simulink model "main_simulation"  (R2025b)
settings: Solver=VariableStepAuto  StartTime=0.0  StopTime=params.sim.duration  MaxStep=params.sim.max_step  MinStep=5  RelTol=0.0001  AbsTol=1e-06
model workspace: external: MAT-File D:\Proiecte Matlab\Cubesat-power-thermal-sim\models\environment\params_simulink.mat (data not in the file)
libraries: fl_lib x5, nesl_utility x4, batteryecm_lib x1
settings Model: Creator=romas  LastModifiedBy=Alex

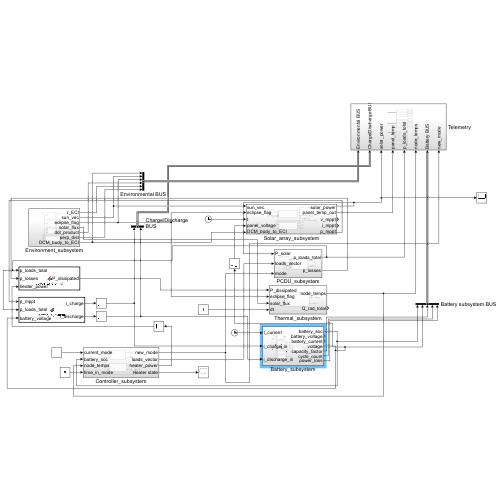
[thumbnail: Simulink's stored preview of the top-level diagram]
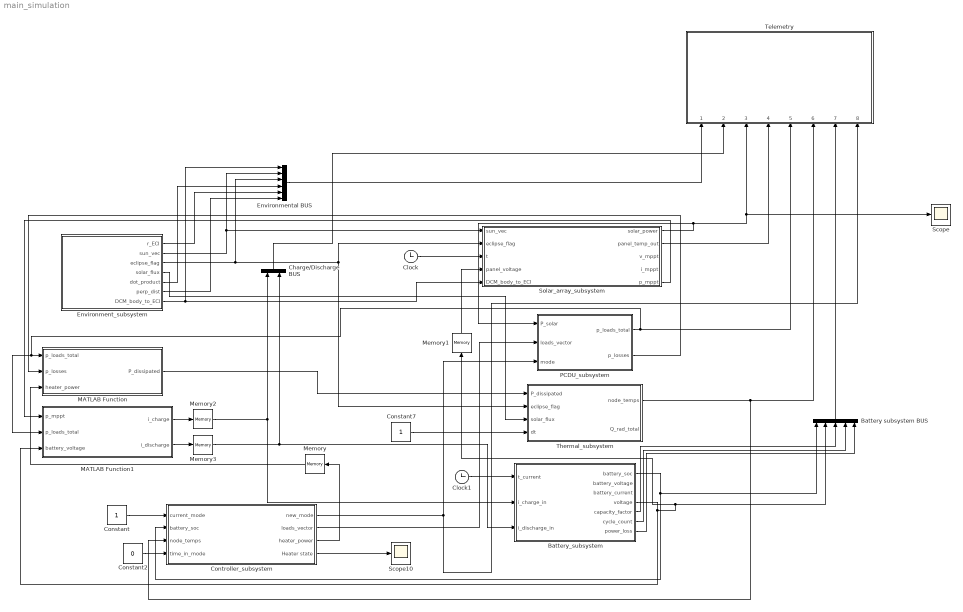
== system main_simulation ==
  Battery subsystem BUS : BusCreator  Inputs=5
  Battery_subsystem : Subsystem
  "Charge/Discharge BUS " : BusCreator  Inputs=2
  Clock : Clock
  Clock1 : Clock
  Constant : Constant
  Constant2 : Constant  Value=0
  Constant7 : Constant
  Controller_subsystem : Subsystem
  Environment_subsystem : Subsystem
  Environmental BUS : BusCreator  Inputs=6
  MATLAB Function : MATLAB Function  TreatAsAtomicUnit=on
  MATLAB Function1 : MATLAB Function  TreatAsAtomicUnit=on
  Memory : Memory
  Memory1 : Memory  InitialCondition=28.8
  Memory2 : Memory
  Memory3 : Memory
  PCDU_subsystem : Subsystem
  Scope : Scope
      settings: ActiveDisplayYMinimum=37.40655674776653  ActiveDisplayYMaximum=42.776597227384748
  Scope10 : Scope
      settings: ActiveDisplayYMinimum=-0.35419792033416531  ActiveDisplayYMaximum=1.2278549732412836  DataLoggingVariableName=ScopeData10
  Solar_array_subsystem : Subsystem
  Telemetry : Subsystem
  Thermal_subsystem : Subsystem
  wires:
  Environment_subsystem/2(sun_vec) -> Solar_array_subsystem/1(sun_vec), Environmental BUS/2
  Environment_subsystem/3(eclipse_flag) -> Environmental BUS/3, Solar_array_subsystem/2(eclipse_flag), Thermal_subsystem/2(eclipse_flag)
  Environment_subsystem/4(solar_flux) -> Thermal_subsystem/3(solar_flux)
  Solar_array_subsystem/1(solar_power) -> PCDU_subsystem/1(P_solar), Scope/1, Telemetry/3(solar_power)
  Constant2/1 -> Controller_subsystem/4(time_in_mode)
  Controller_subsystem/3(heater_power) -> Memory/1
  Controller_subsystem/1(new_mode) -> Telemetry/8(new_mode), PCDU_subsystem/3(mode)
  Controller_subsystem/2(loads_vector) -> PCDU_subsystem/2(loads_vector)
  Battery_subsystem/1(battery_soc) -> Controller_subsystem/2(battery_soc), Battery subsystem BUS/1
  MATLAB Function/1(P_dissipated) -> Thermal_subsystem/1(P_dissipated)
  PCDU_subsystem/1(p_loads_total) -> MATLAB Function1/2(p_loads_total), MATLAB Function/1(p_loads_total), Telemetry/5(p_loads_total)
  PCDU_subsystem/2(p_losses) -> MATLAB Function/2(p_losses)
  Constant7/1 -> Thermal_subsystem/4(dt)
  Memory/1 -> MATLAB Function/3(heater_power)
  Thermal_subsystem/1(node_temps) -> Controller_subsystem/3(node_temps), Telemetry/6(node_temps)
  MATLAB Function1/1(i_charge) -> Memory2/1
  MATLAB Function1/2(i_discharge) -> Memory3/1
  Memory3/1 -> Battery_subsystem/3(i_discharge_in), "Charge/Discharge BUS "/2
  Clock/1 -> Solar_array_subsystem/3(t)
  Clock1/1 -> Battery_subsystem/1(t_current)
  Battery_subsystem/4(voltage) -> Memory1/1, Battery subsystem BUS/2, MATLAB Function1/3(battery_voltage)
  Memory1/1 -> Solar_array_subsystem/4(panel_voltage)
  Memory2/1 -> Battery_subsystem/2(i_charge_in), "Charge/Discharge BUS "/1
  Solar_array_subsystem/2(panel_temp_out) -> Telemetry/4(panel_temp)
  Battery_subsystem/5(capacity_factor) -> Battery subsystem BUS/3
  Battery_subsystem/6(cycle_count) -> Battery subsystem BUS/4
  Battery_subsystem/7(power_loss) -> Battery subsystem BUS/5
  Battery subsystem BUS/1 -> Telemetry/7(Battery BUS)
  Controller_subsystem/4(Heater state) -> Scope10/1
  Environment_subsystem/5(dot_product) -> Environmental BUS/4
  Environment_subsystem/1(r_ECI) -> Environmental BUS/5
  Environment_subsystem/6(perp_dist) -> Environmental BUS/6
  Environmental BUS/1 -> Telemetry/1(Environmental BUS)
  "Charge/Discharge BUS "/1 -> Telemetry/2(Charge/Discharge BUS)
  Environment_subsystem/7(DCM_body_to_ECI) -> Environmental BUS/1, Solar_array_subsystem/5(DCM_body_to_ECI)
  Constant/1 -> Controller_subsystem/1(current_mode)
  Solar_array_subsystem/5(p_mppt) -> MATLAB Function1/1(p_mppt)

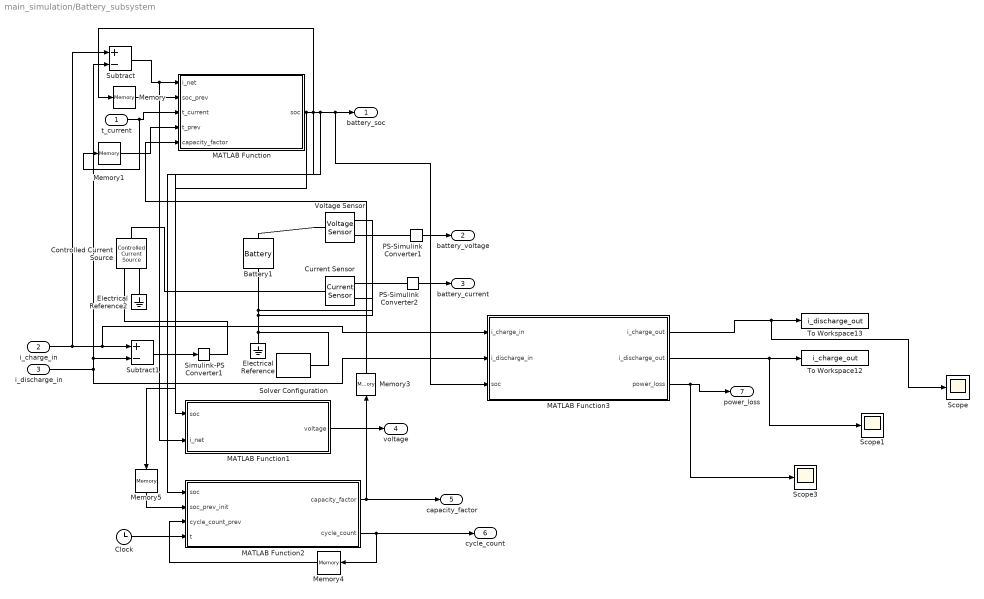
== system main_simulation/Battery_subsystem ==
  t_current : Inport
  i_charge_in : Inport  Port=2
  i_discharge_in : Inport  Port=3
  Battery1 : batteryecm_lib/Battery  Vnom=14.4 V  prm_dir=simscape.enum.battery.prm_dir.disabled  R1_dis=2 Ohm  R1_ch=2 Ohm  R1=0.08 Ohm  prm_AH=simscape.enum.battery.prm_AH.infinite  AH=13.6 A*hr  V1=25.2 V  AH1=2.7 A*hr  prm_R2=simscape.enum.battery.prm_R2.disabled  R2=2000 Ohm  Tmeas=298.15 K  charge_measurement_port=simscape.enum.battery.enable.no  prm_dyn=simscape.enum.battery.prm_dyn.off  Rp1=0.005 Ohm  tau1=30 s  Rp2=0.005 Ohm  tau2=30 s  Rp3=0.005 Ohm  tau3=30 s  Rp4=0.005 Ohm  tau4=30 s  Rp5=0.005 Ohm  tau5=30 s  prm_fade=simscape.enum.battery.prm_fade.disabled  N_fade=100  AH_fade=45 A*hr  R1_fade=2.02 Ohm  R1_ch_fade=2.02 Ohm  V1_fade=10.35 V  prm_age=simscape.enum.battery.prm_age.disabled  prm_age_OCV=simscape.enum.battery.prm_age_OCV.OCV  OCV_age=0.9  SOC_age=60  Tmeas_age=298.15 K  delta_time_age_vec=[0] d  temperature_age_vec=[273] K  OCV_scaling_age=2.2134e6  OCV_offset_age=1.632e6  temp_exp_age=0.515833569 V  t_exp_age=0.75  Vnom_T2=12 V  R1_T2=2.2 Ohm  R1_T2_dis=2.2 Ohm  R1_T2_ch=2.2 Ohm  V1_T2=11.4 V  R2_T2=2200 Ohm  Rp1_T2=0.005 Ohm  tau1_T2=30 s  Rp2_T2=0.005 Ohm  tau2_T2=30 s  Rp3_T2=0.005 Ohm  tau3_T2=30 s  Rp4_T2=0.005 Ohm  tau4_T2=30 s  Rp5_T2=0.005 Ohm  tau5_T2=30 s  Tmeas2=273.15 K  thermal_port=simscape.enum.thermaleffects.omit  thermal_mass=30000 J/K  i_specify=off  i_priority=None  i=0 A  i_nominal_specify=off  i_nominal_value=1  i_nominal_unit=A  v_specify=off  v_priority=None  v=0 V  v_nominal_specify=off  v_nominal_value=1  v_nominal_unit=V  charge_specify=off  charge_priority=High  charge=50 A*hr  charge_nominal_specify=off  charge_nominal_value=1  charge_nominal_unit=A*hr  num_cycles_specify=off  num_cycles_priority=High  num_cycles=0  num_cycles_nominal_specify=off  num_cycles_nominal_value=1  num_cycles_nominal_unit=1  temperature_specify=off  temperature_priority=High  temperature=298.15 K  temperature_nominal_specify=off  temperature_nominal_value=1  temperature_nominal_unit=K
  Clock : Clock
  Controlled Current Source : fl_lib/Electrical/Electrical Sources/Controlled Current Source
      settings: LogSimulationData=on
  Current Sensor : fl_lib/Electrical/Electrical Sensors/Current Sensor
  Electrical Reference : fl_lib/Electrical/Electrical Elements/Electrical Reference
  Electrical Reference2 : fl_lib/Electrical/Electrical Elements/Electrical Reference
  MATLAB Function : MATLAB Function  TreatAsAtomicUnit=on
  MATLAB Function1 : MATLAB Function  TreatAsAtomicUnit=on
  MATLAB Function2 : MATLAB Function  TreatAsAtomicUnit=on
  MATLAB Function3 : MATLAB Function  TreatAsAtomicUnit=on
  Memory : Memory  InitialCondition=0.5
  Memory1 : Memory
  Memory3 : Memory  InitialCondition=1
  Memory4 : Memory
  Memory5 : Memory  InitialCondition=0.5
  PS-Simulink Converter1 : nesl_utility/PS-Simulink Converter  PhysicalDomain=network_engine_domain  SubClassName=ps_output  LeftPortType=input  RightPortType=output  PseudoPeriodic=off  Frequencies=[]  VectorFormat=inherit  Unit=inherit  AffineConversion=off
  PS-Simulink Converter2 : nesl_utility/PS-Simulink Converter  PhysicalDomain=network_engine_domain  SubClassName=ps_output  LeftPortType=input  RightPortType=output  PseudoPeriodic=off  Frequencies=[]  VectorFormat=inherit  Unit=inherit  AffineConversion=off
  Scope : Scope
      settings: ActiveDisplayYMinimum=1.0175731701322981  ActiveDisplayYMaximum=4.0182844452187787  DataLoggingVariableName=ScopeData6
  Scope1 : Scope
      settings: ActiveDisplayYMinimum=-0.49399999999999988  ActiveDisplayYMaximum=4.446  DataLoggingVariableName=ScopeData8
  Scope3 : Scope
      settings: ActiveDisplayYMinimum=-7.2208170321005092  ActiveDisplayYMaximum=9.8697764484998771  DataLoggingVariableName=ScopeData11
  Simulink-PS Converter1 : nesl_utility/Simulink-PS Converter  PhysicalDomain=network_engine_domain  SubClassName=ps_input  LeftPortType=input  RightPortType=output  PseudoPeriodic=off  Frequencies=[]  NoiseDistribution=none  NoiseParameters=[]  Unit=1  AffineConversion=off  FilteringAndDerivatives=provide  SimscapeFilterOrder=1  InputFilterTimeConstant=0.001  UdotUserProvided=0
  Solver Configuration : nesl_utility/Solver Configuration  PhysicalDomain=network_engine_domain  SubClassName=solver  LeftPortType=input  RightPortType=generic  Tones=[]  Harmonics=[]  SimulateNoise=off  Profile=off  UseLocalSampling=off  EnableSwitchedLinearOptims=on  FrequencyDomain=off  UseCCode=off  RelTol=0.001  AbsTol=0.001  MinStep=1e-09  ToWorkspace=off  RevertToSquareIcSolve=off  NumHomotopyIterations=100  PhasorMode=off  PhasorModeNumHarmonics=1  ConsistencySolver=NEWTON_XTOL_AFTER_FTOL  IndexReductionMethod=DerivativeReplacement  DoDC=off  ResidualTolerance=1e-09  ConsistencyTolSource=GLOBAL  ConsistencyAbsTol=0.001  ConsistencyRelTol=0.001  ConsistencyTolFactor=0.001  UseLocalSolver=off  LocalSolverChoice=NE_BACKWARD_EULER_ADVANCER  ResolveIndetEquations=on  FunctionEvalNumThread=1  LocalSolverSampleTime=0.001  DoFixedCost=off  MaxNonlinIter=3  MaxModeIter=2  ComputeImpulses=off  ImpulseIterations=2  LinearAlgebra=auto  LinearAlgebraNumThread=0  EquationFormulation=NE_TIME_EF  DelaysMemoryBudget=1024  AutomaticFiltering=on  FilteringTimeConstant=0.001  PartitionStorageMethod=AS_NEEDED  PartitionMemoryBudget=1024  PartitionMethod=ROBUST  MultibodyUseLocalSolver=off  MultibodyLocalSolverChoice=ODE1  MultibodyLocalSolverSampleTime=0.001
  Subtract : Sum  Inputs=+-
  Subtract1 : Sum  Inputs=+-
  To Workspace12 : ToWorkspace  VariableName=i_charge_out  SaveFormat=Timeseries  SampleTime=-1
  To Workspace13 : ToWorkspace  VariableName=i_discharge_out  SaveFormat=Timeseries  SampleTime=-1
  Voltage Sensor : fl_lib/Electrical/Electrical Sensors/Voltage Sensor
  battery_soc : Outport
  battery_voltage : Outport  Port=2
  battery_current : Outport  Port=3
  voltage : Outport  Port=4
  capacity_factor : Outport  Port=5
  cycle_count : Outport  Port=6
  power_loss : Outport  Port=7
  wires:
  MATLAB Function/1(soc) -> MATLAB Function1/1(soc), Memory5/1, Memory/1, MATLAB Function3/3(soc), battery_soc/1, MATLAB Function2/1(soc)
  Subtract1/1 -> Simulink-PS Converter1/1
  PS-Simulink Converter2/1 -> battery_current/1
  PS-Simulink Converter1/1 -> battery_voltage/1
  t_current/1 -> MATLAB Function/3(t_current), Memory1/1
  Memory1/1 -> MATLAB Function/4(t_prev)
  MATLAB Function1/1(voltage) -> voltage/1
  MATLAB Function2/1(capacity_factor) -> Memory3/1, capacity_factor/1
  Clock/1 -> MATLAB Function2/4(t)
  Memory3/1 -> MATLAB Function/5(capacity_factor)
  MATLAB Function2/2(cycle_count) -> Memory4/1, cycle_count/1
  Memory4/1 -> MATLAB Function2/3(cycle_count_prev)
  Memory/1 -> MATLAB Function/2(soc_prev)
  Memory5/1 -> MATLAB Function2/2(soc_prev_init)
  Subtract/1 -> MATLAB Function1/2(i_net), MATLAB Function/1(i_net)
  i_charge_in/1 -> Subtract/1, MATLAB Function3/1(i_charge_in), Subtract1/1
  i_discharge_in/1 -> MATLAB Function3/2(i_discharge_in), Subtract/2, Subtract1/2
  MATLAB Function3/1(i_charge_out) -> Scope/1, To Workspace13/1
  MATLAB Function3/2(i_discharge_out) -> Scope1/1, To Workspace12/1
  MATLAB Function3/3(power_loss) -> Scope3/1, power_loss/1
  connections:
  Battery1/RConn1 -- Voltage Sensor/RConn2 -- Current Sensor/RConn2 -- Solver Configuration/RConn1 -- Electrical Reference/LConn1
  PS-Simulink Converter1/LConn1 -- Voltage Sensor/RConn1
  PS-Simulink Converter2/LConn1 -- Current Sensor/RConn1
  Simulink-PS Converter1/RConn1 -- Controlled Current Source/RConn1
  Electrical Reference2/LConn1 -- Controlled Current Source/RConn2
  Controlled Current Source/LConn1 -- Current Sensor/LConn1
  Voltage Sensor/LConn1 -- Battery1/LConn1

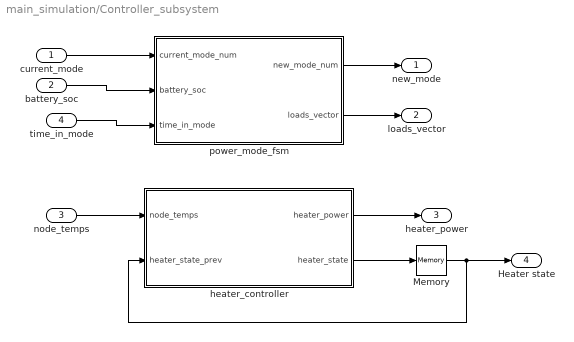
== system main_simulation/Controller_subsystem ==
  current_mode : Inport
  battery_soc : Inport  Port=2
  node_temps : Inport  Port=3
  time_in_mode : Inport  Port=4
  Memory : Memory  InitialCondition=[0;0;0]
  heater_controller : MATLAB Function  TreatAsAtomicUnit=on
  power_mode_fsm : MATLAB Function  TreatAsAtomicUnit=on
  new_mode : Outport
  loads_vector : Outport  Port=2
  heater_power : Outport  Port=3
  Heater state : Outport  Port=4
  wires:
  battery_soc/1 -> power_mode_fsm/2(battery_soc)
  node_temps/1 -> heater_controller/1(node_temps)
  time_in_mode/1 -> power_mode_fsm/3(time_in_mode)
  heater_controller/2(heater_state) -> Memory/1
  power_mode_fsm/2(loads_vector) -> loads_vector/1
  heater_controller/1(heater_power) -> heater_power/1
  Memory/1 -> Heater state/1, heater_controller/2(heater_state_prev)
  power_mode_fsm/1(new_mode_num) -> new_mode/1
  current_mode/1 -> power_mode_fsm/1(current_mode_num)

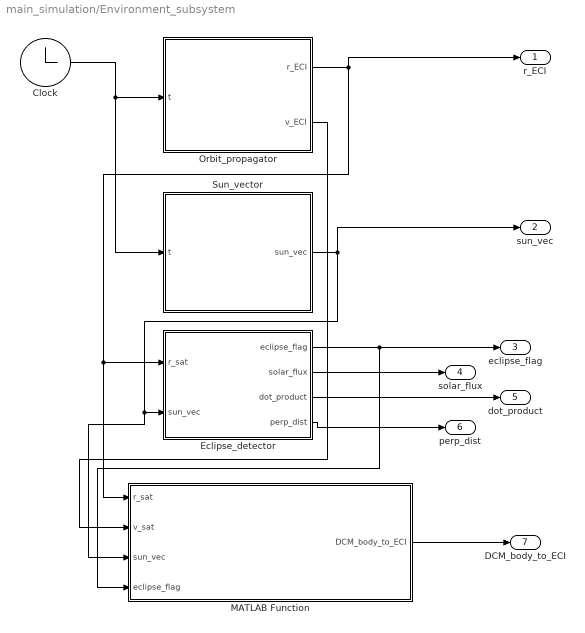
== system main_simulation/Environment_subsystem ==
  Clock : Clock
  Eclipse_detector : MATLAB Function  TreatAsAtomicUnit=on
  MATLAB Function : MATLAB Function  TreatAsAtomicUnit=on
  Orbit_propagator : MATLAB Function  TreatAsAtomicUnit=on
  Sun_vector : MATLAB Function  TreatAsAtomicUnit=on
  r_ECI : Outport
  sun_vec : Outport  Port=2
  eclipse_flag : Outport  Port=3
  solar_flux : Outport  Port=4
  dot_product : Outport  Port=5
  perp_dist : Outport  Port=6
  DCM_body_to_ECI : Outport  Port=7
  wires:
  Clock/1 -> Sun_vector/1(t), Orbit_propagator/1(t)
  Orbit_propagator/1(r_ECI) -> r_ECI/1, MATLAB Function/1(r_sat), Eclipse_detector/1(r_sat)
  Sun_vector/1(sun_vec) -> sun_vec/1, MATLAB Function/3(sun_vec), Eclipse_detector/2(sun_vec)
  Eclipse_detector/1(eclipse_flag) -> MATLAB Function/4(eclipse_flag), eclipse_flag/1
  Eclipse_detector/2(solar_flux) -> solar_flux/1
  Eclipse_detector/3(dot_product) -> dot_product/1
  Eclipse_detector/4(perp_dist) -> perp_dist/1
  Orbit_propagator/2(v_ECI) -> MATLAB Function/2(v_sat)
  MATLAB Function/1(DCM_body_to_ECI) -> DCM_body_to_ECI/1

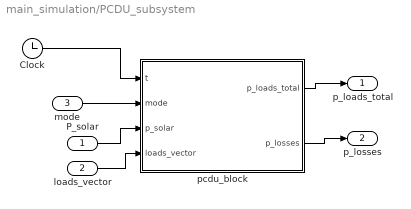
== system main_simulation/PCDU_subsystem ==
  P_solar : Inport
  loads_vector : Inport  Port=2
  mode : Inport  Port=3
  Clock : Clock
  pcdu_block : MATLAB Function  TreatAsAtomicUnit=on
  p_loads_total : Outport
  p_losses : Outport  Port=2
  wires:
  P_solar/1 -> pcdu_block/3(p_solar)
  loads_vector/1 -> pcdu_block/4(loads_vector)
  pcdu_block/2(p_losses) -> p_losses/1
  pcdu_block/1(p_loads_total) -> p_loads_total/1
  Clock/1 -> pcdu_block/1(t)
  mode/1 -> pcdu_block/2(mode)

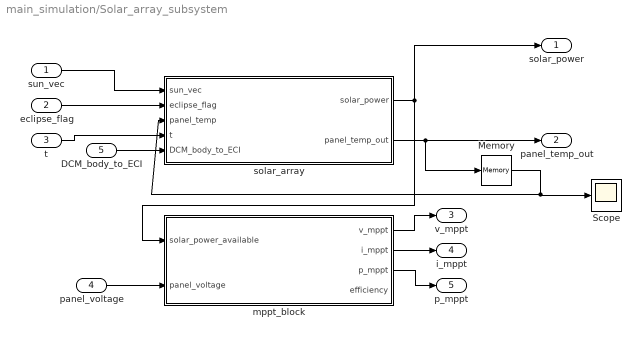
== system main_simulation/Solar_array_subsystem ==
  sun_vec : Inport
  eclipse_flag : Inport  Port=2
  t : Inport  Port=3
  panel_voltage : Inport  Port=4
  DCM_body_to_ECI : Inport  Port=5
  Memory : Memory  InitialCondition=301
  Scope : Scope
      settings: ActiveDisplayYMinimum=223.83654185066587  ActiveDisplayYMaximum=445.32686737029553
  mppt_block : MATLAB Function  TreatAsAtomicUnit=on
  solar_array : MATLAB Function  TreatAsAtomicUnit=on
  solar_power : Outport
  panel_temp_out : Outport  Port=2
  v_mppt : Outport  Port=3
  i_mppt : Outport  Port=4
  p_mppt : Outport  Port=5
  wires:
  Memory/1 -> Scope/1, solar_array/3(panel_temp)
  solar_array/1(solar_power) -> solar_power/1, mppt_block/1(solar_power_available)
  sun_vec/1 -> solar_array/1(sun_vec)
  eclipse_flag/1 -> solar_array/2(eclipse_flag)
  t/1 -> solar_array/4(t)
  panel_voltage/1 -> mppt_block/2(panel_voltage)
  mppt_block/2(i_mppt) -> i_mppt/1
  mppt_block/1(v_mppt) -> v_mppt/1
  mppt_block/3(p_mppt) -> p_mppt/1
  solar_array/2(panel_temp_out) -> Memory/1, panel_temp_out/1
  DCM_body_to_ECI/1 -> solar_array/5(DCM_body_to_ECI)

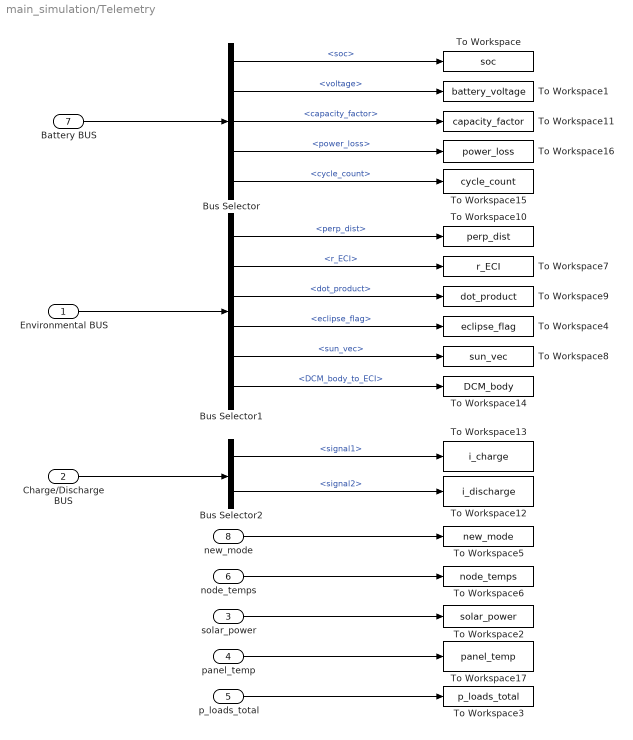
== system main_simulation/Telemetry ==
  Environmental BUS : Inport
  Charge/Discharge BUS : Inport  Port=2
  solar_power : Inport  Port=3
  panel_temp : Inport  Port=4
  p_loads_total : Inport  Port=5
  node_temps : Inport  Port=6
  Battery BUS : Inport  Port=7
  new_mode : Inport  Port=8
  Bus Selector : BusSelector  OutputSignals=soc,voltage,capacity_factor,power_loss,cycle_count
  Bus Selector1 : BusSelector  OutputSignals=perp_dist,r_ECI,dot_product,eclipse_flag,sun_vec,DCM_body_to_ECI
  Bus Selector2 : BusSelector  OutputSignals=signal1,signal2
  To Workspace : ToWorkspace  VariableName=soc  SaveFormat=Timeseries  SampleTime=-1
  To Workspace1 : ToWorkspace  VariableName=battery_voltage  SaveFormat=Timeseries  SampleTime=-1
  To Workspace10 : ToWorkspace  VariableName=perp_dist  SaveFormat=Timeseries  SampleTime=-1
  To Workspace11 : ToWorkspace  VariableName=capacity_factor  SaveFormat=Timeseries  SampleTime=-1
  To Workspace12 : ToWorkspace  VariableName=i_discharge  SaveFormat=Timeseries  SampleTime=-1
  To Workspace13 : ToWorkspace  VariableName=i_charge  SaveFormat=Timeseries  SampleTime=-1
  To Workspace14 : ToWorkspace  VariableName=DCM_body  SaveFormat=Timeseries  SampleTime=-1
  To Workspace15 : ToWorkspace  VariableName=cycle_count  SaveFormat=Timeseries  SampleTime=-1
  To Workspace16 : ToWorkspace  VariableName=power_loss  SaveFormat=Timeseries  SampleTime=-1
  To Workspace17 : ToWorkspace  VariableName=panel_temp  SaveFormat=Timeseries  SampleTime=-1
  To Workspace2 : ToWorkspace  VariableName=solar_power  SaveFormat=Timeseries  SampleTime=-1
  To Workspace3 : ToWorkspace  VariableName=p_loads_total  SaveFormat=Timeseries  SampleTime=-1
  To Workspace4 : ToWorkspace  VariableName=eclipse_flag  SaveFormat=Timeseries  SampleTime=-1
  To Workspace5 : ToWorkspace  VariableName=new_mode  SaveFormat=Timeseries  SampleTime=-1
  To Workspace6 : ToWorkspace  VariableName=node_temps  SaveFormat=Timeseries  SampleTime=-1
  To Workspace7 : ToWorkspace  VariableName=r_ECI  SaveFormat=Timeseries  SampleTime=-1
  To Workspace8 : ToWorkspace  VariableName=sun_vec  SaveFormat=Timeseries  SampleTime=-1
  To Workspace9 : ToWorkspace  VariableName=dot_product  SaveFormat=Timeseries  SampleTime=-1
  wires:
  Battery BUS/1 -> Bus Selector/1
  Bus Selector/1 -> To Workspace/1  "<soc>"
  Bus Selector/2 -> To Workspace1/1  "<voltage>"
  Bus Selector/3 -> To Workspace11/1  "<capacity_factor>"
  Bus Selector/4 -> To Workspace16/1  "<power_loss>"
  Bus Selector/5 -> To Workspace15/1  "<cycle_count>"
  Environmental BUS/1 -> Bus Selector1/1
  Bus Selector1/1 -> To Workspace10/1  "<perp_dist>"
  Bus Selector1/2 -> To Workspace7/1  "<r_ECI>"
  Bus Selector1/3 -> To Workspace9/1  "<dot_product>"
  Bus Selector1/4 -> To Workspace4/1  "<eclipse_flag>"
  Bus Selector1/5 -> To Workspace8/1  "<sun_vec>"
  Charge/Discharge BUS/1 -> Bus Selector2/1
  Bus Selector2/1 -> To Workspace13/1  "<signal1>"
  Bus Selector2/2 -> To Workspace12/1  "<signal2>"
  new_mode/1 -> To Workspace5/1
  node_temps/1 -> To Workspace6/1
  solar_power/1 -> To Workspace2/1
  panel_temp/1 -> To Workspace17/1
  p_loads_total/1 -> To Workspace3/1
  Bus Selector1/6 -> To Workspace14/1  "<DCM_body_to_ECI>"

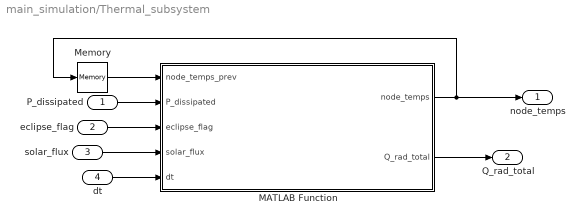
== system main_simulation/Thermal_subsystem ==
  P_dissipated : Inport
  eclipse_flag : Inport  Port=2
  solar_flux : Inport  Port=3
  dt : Inport  Port=4
  MATLAB Function : MATLAB Function  TreatAsAtomicUnit=on
  Memory : Memory  InitialCondition=293.15 * ones(12,1)
  node_temps : Outport
  Q_rad_total : Outport  Port=2
  wires:
  Memory/1 -> MATLAB Function/1(node_temps_prev)
  MATLAB Function/1(node_temps) -> node_temps/1, Memory/1
  MATLAB Function/2(Q_rad_total) -> Q_rad_total/1
  solar_flux/1 -> MATLAB Function/4(solar_flux)
  eclipse_flag/1 -> MATLAB Function/3(eclipse_flag)
  P_dissipated/1 -> MATLAB Function/2(P_dissipated)
  dt/1 -> MATLAB Function/5(dt)

== matlab function main_simulation/PCDU_subsystem/pcdu_block ==
  data: t input; mode input; p_solar input; p_loads_total output; loads_vector input; p_losses output; params parameter
function [p_loads_total, p_losses] = pcdu_block(t, mode, p_solar, loads_vector, params)
    p_loads_total = 0;
    p_losses = 0;
    
    p_obc_base = params.loads.obc.power_avg;
    p_pcdu_idle = params.pcdu.quiescent_power;
    
    orbit_period = params.orbit.period;
    orbit_phase = mod(t, orbit_period) / orbit_period;
    
    %ADCS: active 70% of orbit
    if loads_vector(2) > 0
        if orbit_phase < 0.70
            p_adcs = params.loads.adcs.power_peak;
        else
            p_adcs = params.loads.adcs.power_avg * 0.2;
        end
    else
        p_adcs = 0;
    end
    
    %COMMS: bursts every 6 hours for 10 min
    if loads_vector(3) > 0
        pass_period = 14400;
        pass_duration = 600;
        time_in_pass = mod(t, pass_period);
        
        if time_in_pass < pass_duration
            p_comms = params.loads.comms.power_peak;
        else
            p_comms = params.loads.comms.power_avg;
        end
    else
        p_comms = 0;
    end
    
    %PAYLOAD: active 25% of orbit in science mode
    %MODE: 0=safe, 1=nominal, 2=science
    if loads_vector(4) > 0 && mode == 2  % CHANGED FROM mode==3
        if orbit_phase > 0.35 && orbit_phase < 0.60
            p_payload = params.loads.payload.power_peak;
        else
            p_payload = 0;
        end
    else
        p_payload = 0;
    end
    
    %Total
    p_loads_total = p_obc_base + p_pcdu_idle + p_adcs + p_comms + p_payload;
    
    %Clamp to mode budget
    %MODE: 0=safe, 1=nominal, 2=science
    if mode == 0  % CHANGED FROM case 1
        p_loads_total = min(p_loads_total, params.power_mode.safe.power_budget);
    elseif mode == 1  % CHANGED FROM case 2
        p_loads_total = min(p_loads_total, params.power_mode.nominal.power_budget);
    elseif mode == 2  % CHANGED FROM case 3
        p_loads_total = min(p_loads_total, params.power_mode.science.power_budget);
    end
    
    %PCDU losses
    efficiency = 0.95;
    p_losses = p_loads_total * (1 - efficiency) / efficiency;
end

== matlab function main_simulation/Thermal_subsystem/MATLAB Function ==
  data: node_temps_prev input; node_temps output; P_dissipated input; eclipse_flag input; solar_flux input; dt input; Q_rad_total output; params parameter
function [node_temps, Q_rad_total] = thermal_model_block(node_temps_prev, P_dissipated, eclipse_flag, solar_flux, dt, params)
    %Simplified 12-node thermal model
    %node_temps_prev: previous temps [K] (12x1)
    %P_dissipated: power dissipated at each node [W] (12x1) 
    %eclipse_flag: boolean
    %solar_flux: W/m^2
    
    %Thermal masses [J/K]
    C = [1600; 120; 200; 300; 150; 250; 1800; 100; 100; 150; 150; 80];
    
    %Conductance matrix [W/K] - from params
    G = zeros(12,12);
    G(1,7) = 2.5; G(7,1) = 2.5; %Battery-Structure
    G(2,7) = 0.8; G(7,2) = 0.8; %Solar-Structure
    G(3,7) = 3.0; G(7,3) = 3.0; %OBC-Structure
    G(4,7) = 2.8; G(7,4) = 2.8; %ADCS-Structure
    G(5,7) = 2.5; G(7,5) = 2.5; %COMMS-Structure
    G(6,7) = 3.2; G(7,6) = 3.2; %Payload-Structure
    G(7,8) = 4.0; G(8,7) = 4.0; %Structure-RadXp
    G(7,9) = 4.0; G(9,7) = 4.0; %Structure-RadXm
    G(7,10) = 5.0; G(10,7) = 5.0; %Structure-RadYp
    G(7,11) = 5.0; G(11,7) = 5.0; %Structure-RadYm
    G(7,12) = 6.0; G(12,7) = 6.0; %Structure-RadZp
    
    %Conduction heat flows
    Q_cond = zeros(12,1);
    for i = 1:12
        for j = 1:12
            if G(i,j) > 0
                Q_cond(i) = Q_cond(i) + G(i,j) * (node_temps_prev(j) - node_temps_prev(i));
            end
        end
    end
    
    %Radiation to space (Stefan-Boltzmann)
    sigma = 5.670374419e-8; % W/m^2/K^4
    epsilon = 0.90; % Radiator emissivity
    A_rad = [0; 0; 0; 0; 0; 0; 0; 0.0828; 0.0828; 0.0366; 0.0366; 0.0226]; %Radiator areas
    Q_rad = -sigma * epsilon * A_rad .* (node_temps_prev.^4);
    Q_rad_total = sum(Q_rad);
    
    %Net heat flow
    Q_net = P_dissipated + Q_cond + Q_rad;
    
    %Temperature update (Euler integration)
    dT = (Q_net ./ C) * dt;
    node_temps = node_temps_prev + dT;
    
    %Clamp to physical range
    node_temps = max(200, min(400, node_temps));
end

== matlab function main_simulation/MATLAB Function ==
  data: p_loads_total input; P_dissipated output; p_losses input; heater_power input
function P_dissipated = power_to_thermal(p_loads_total, p_losses, heater_power)
       %Map to 12 nodes: [Battery, Solar, OBC, ADCS, COMMS, Payload, Structure, RadXp, RadXm, RadYp, RadYm, RadZp]
       P_dissipated = zeros(12,1);
       P_dissipated(1) = heater_power * 0.67; %Battery heater 
       P_dissipated(3) = p_loads_total * 0.15 + heater_power * 0.08; %OBC + heater
       P_dissipated(4) = p_loads_total * 0.48; %ADCS
       P_dissipated(5) = p_loads_total * 0.36; %COMMS
       P_dissipated(6) = p_loads_total * 0.01 + heater_power * 0.25; %Payload + heater
       P_dissipated(7) = p_losses; %PCDU losses in structure
   end

== matlab function main_simulation/MATLAB Function1 ==
  data: p_mppt input; i_charge output; p_loads_total input; battery_voltage input; i_discharge output; params parameter
function [i_charge, i_discharge] = power_to_current(p_mppt, p_loads_total, battery_voltage, params)
    %Protect against zero/low voltage
    battery_voltage = max(battery_voltage, params.pcdu.bus_voltage_min); 
    
    i_charge = (p_mppt * params.pcdu.efficiency_mppt) / battery_voltage; %i_mppt;
    i_discharge = p_loads_total / battery_voltage;
    
    i_charge = max(0, min(i_charge, params.pcdu.current_max / 2));
    i_discharge = max(0, min(i_discharge, params.pcdu.current_max / 2));
end

== matlab function main_simulation/Environment_subsystem/MATLAB Function ==
  data: r_sat input; DCM_body_to_ECI output size=[3 3]; v_sat input size=[3 1]; sun_vec input size=[3 1]; eclipse_flag input size=[1 1]; params parameter
function DCM_body_to_ECI  = attitude_determination_block(r_sat, v_sat, sun_vec, eclipse_flag, params)
    [DCM_body_to_ECI] = attitude_determination(r_sat, v_sat, sun_vec, eclipse_flag, params);
end

== matlab function main_simulation/Battery_subsystem/MATLAB Function1 ==
  data: soc input; voltage output; i_net input; params parameter
function voltage = battery_voltage_block(soc, i_net, params)
    voltage = battery_voltage_model(soc, i_net, params);
end

== matlab function main_simulation/Battery_subsystem/MATLAB Function2 ==
  data: soc input; capacity_factor output; soc_prev_init input; cycle_count_prev input; t input; cycle_count output; params parameter
function [capacity_factor, cycle_count] = fcn(soc, soc_prev_init, cycle_count_prev, t, params)

persistent last_cycle_t;

% Reset on t=0 fixes multi-run caching
if isempty(last_cycle_t) || t == 0
    last_cycle_t = 0;
end

%% Calendar aging — Arrhenius + SEI growth
mission_years  = t / (365.25 * 86400);
T_bat  = params.battery.temp_nominal;
T_ref  = 298.15;
Ea     = 24000;
R_gas  = 8.314;
temp_accel         = exp((Ea/R_gas) * (1/T_ref - 1/T_bat));
bulk_fade          = exp(-params.battery.calendar_fade_rate * mission_years * temp_accel);
k_sei              = 0.004;
sei_fade           = min(0.15, k_sei * sqrt(mission_years * temp_accel));
calendar_retention = bulk_fade * (1 - sei_fade);
calendar_retention = max(0.5, calendar_retention);

%% Cycle counting — one Woehler-weighted cycle per orbit period
% Avoids noise-driven false reversals from 50s solver steps
orbit_period    = params.orbit.period;
cycle_increment = 0;

if t - last_cycle_t >= orbit_period
    dod_actual      = params.battery.SOC_max - params.battery.SOC_min;  % ~0.20
    dod_rated       = 0.25;
    k_wohler        = 1.5;
    cycle_increment = (dod_actual / dod_rated)^k_wohler;
    last_cycle_t    = t;
end

cycle_count = cycle_count_prev + cycle_increment;

%% Cycle-life fade
cycle_retention = 1.0 - 0.20 * (cycle_count / params.battery.cycle_life);
cycle_retention = max(0.5, cycle_retention);

%% Combined
capacity_factor = calendar_retention * cycle_retention;
capacity_factor = max(0.5, min(1.0, capacity_factor));

end

== matlab function main_simulation/Battery_subsystem/MATLAB Function3 ==
  data: i_charge_in input; i_charge_out output; i_discharge_in input; soc input; i_discharge_out output; power_loss output; params parameter
function [i_charge_out, i_discharge_out, power_loss] = battery_efficiency(i_charge_in, i_discharge_in, soc, params)
%Get efficiency from params

i_charge_in    = max(0, i_charge_in);
i_discharge_in = max(0, i_discharge_in);

eta_charge = params.pcdu.efficiency_battery_charge;  % 0.95

%Discharge efficiency based on C-rate
c_rate = i_discharge_in / params.battery.capacity;

if c_rate < 0.1
    eta_discharge = 0.99;
elseif c_rate < 0.5
    eta_discharge = 0.97;
else
    eta_discharge = 0.95;
end

%Apply efficiencies
i_charge_out = i_charge_in * eta_charge;
i_discharge_out = i_discharge_in;  % Load current unchanged

%Power loss
V_nom = params.battery.nominal_voltage;
power_loss = i_charge_in * V_nom * (1 - eta_charge) + ...
             i_discharge_in * V_nom * (1 - eta_discharge);

end

== matlab function main_simulation/Environment_subsystem/Sun_vector ==
  data: t input; sun_vec output; params parameter
function sun_vec = sun_vector_block(t, params)
    sun_vec = sun_vector(t, params);
end

== matlab function main_simulation/Environment_subsystem/Orbit_propagator ==
  data: t input; r_ECI output; v_ECI output; params parameter
function [r_ECI, v_ECI] = orbit_propagator_block(t, params)
    %params is now a Parameter (from Model Workspace), not an input
    [r_ECI, v_ECI] = orbit_propagator(t, params);
end

== matlab function main_simulation/Environment_subsystem/Eclipse_detector ==
  data: r_sat input; sun_vec input; eclipse_flag output; solar_flux output; dot_product output; perp_dist output; params parameter
function [eclipse_flag, solar_flux, dot_product, perp_dist] = eclipse_detector_block(r_sat, sun_vec, params)
    [eclipse_flag, solar_flux] = eclipse_detector(r_sat, sun_vec, params);
    
    %Calculate perpendicular distance (copy logic from eclipse_detector.m)
    proj_length = dot(r_sat, sun_vec);
    proj_point = proj_length * sun_vec;
    perp_vec = r_sat - proj_point;
    perp_dist = norm(perp_vec);
    
    dot_product = dot(r_sat, sun_vec);
end

== matlab function main_simulation/Solar_array_subsystem/solar_array ==
  data: sun_vec input size=[3 1]; solar_power output; eclipse_flag input size=[1 1]; panel_temp input size=[1 1]; t input size=[1 1]; DCM_body_to_ECI input; panel_temp_out output; params parameter
function [solar_power, panel_temp_out]  = solar_array_block(sun_vec, eclipse_flag, panel_temp, t, DCM_body_to_ECI,  params)
    [solar_power, panel_temp_out] = solar_array_model(sun_vec, eclipse_flag, panel_temp, t, DCM_body_to_ECI, params);
end

== matlab function main_simulation/Solar_array_subsystem/mppt_block ==
  data: solar_power_available input; v_mppt output; panel_voltage input; i_mppt output; p_mppt output; efficiency output; params parameter
function [v_mppt, i_mppt, p_mppt, efficiency] = mppt_block(solar_power_available, panel_voltage, params)
    [v_mppt, i_mppt, p_mppt, efficiency] = mppt_algorithm(solar_power_available, panel_voltage, params);
end

== matlab function main_simulation/Controller_subsystem/power_mode_fsm ==
  data: current_mode_num input; new_mode_num output; battery_soc input; time_in_mode input; loads_vector output; params parameter
function [new_mode_num, loads_vector] = power_mode_fsm_block(current_mode_num, battery_soc, time_in_mode, params)
    %MODE NUMBERING: 0=safe, 1=nominal, 2=science
    %Convert numeric to string
    
    modes = {'safe', 'nominal', 'science'};
    current_mode = modes{current_mode_num + 1};  % +1 because MATLAB arrays are 1-indexed
    
    [new_mode, loads_enabled] = power_mode_fsm(current_mode, battery_soc, time_in_mode, params);
    
    %Convert string back to numeric (0/1/2)
    if strcmp(new_mode, 'safe')
        new_mode_num = 0;
    elseif strcmp(new_mode, 'nominal')
        new_mode_num = 1;
    else  %'science'
        new_mode_num = 2;
    end
    
    %Convert cell array to boolean vector [OBC, ADCS, COMMS, Payload]
    loads_vector = [false; false; false; false];
    for i = 1:length(loads_enabled)
        switch loads_enabled{i}
            case 'obc'
                loads_vector(1) = true;
            case 'adcs'
                loads_vector(2) = true;
            case 'comms'
                loads_vector(3) = true;
            case 'payload'
                loads_vector(4) = true;
        end
    end
end

== matlab function main_simulation/Controller_subsystem/heater_controller ==
  data: node_temps input; heater_power output; heater_state_prev input; heater_state output; params parameter
function [heater_power, heater_state] = heater_controller_block(node_temps, heater_state_prev, params)
    [heater_power, heater_state] = heater_controller(node_temps, heater_state_prev, params);
end

== matlab function main_simulation/Battery_subsystem/MATLAB Function ==
  data: i_net input; soc output; soc_prev input; t_current input; t_prev input; capacity_factor input; params parameter
function soc = battery_soc_tracker(i_net, soc_prev, t_current, t_prev, capacity_factor, params)
    Q_nominal = params.battery.capacity; % Ah
    Q_effective = Q_nominal * capacity_factor;  % Apply degradation
    dt = t_current - t_prev;
    dt = max(dt, 0.001);
    dSOC = (i_net * dt) / (Q_effective * 3600);
    soc = soc_prev + dSOC;
    soc = max(params.battery.SOC_min, min(params.battery.SOC_max, soc));
end
